simulink model "dc_motor"  (R2025a)
settings: Solver=ode45  StartTime=0.0  StopTime=2  RelTol=1e-3
InitFcn:
  | motor_parameters;
values from neighbouring files (symbols this model uses):
  b = 1e-4    (= 0.0001)    [motor_parameters.m]
  J = 1e-4    (= 0.0001)    [motor_parameters.m]
  Ke = 0.05    [motor_parameters.m]
  Kt = 0.05    [motor_parameters.m]
  L = 0.005    [motor_parameters.m]
  R = 2.0    (= 2)    [motor_parameters.m]
  T_load = 0.01    [motor_parameters.m]
  T_step_time = 0.5    [motor_parameters.m]
  Ts_plant = 0.001    [motor_parameters.m]
  V_step_time = 0.1    [motor_parameters.m]
  V_supply = 6.0    (= 6)    [motor_parameters.m]
undefined symbols (not defined in the file or in its folder): DiscIntNeverNeededParam
settings Model: Creator=quan  LastModifiedBy=quan

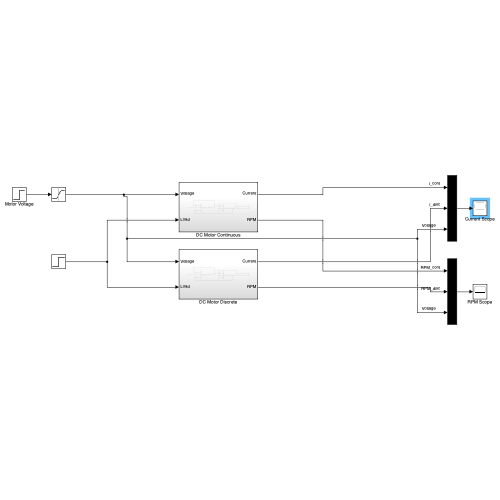
[thumbnail: Simulink's stored preview of the top-level diagram]
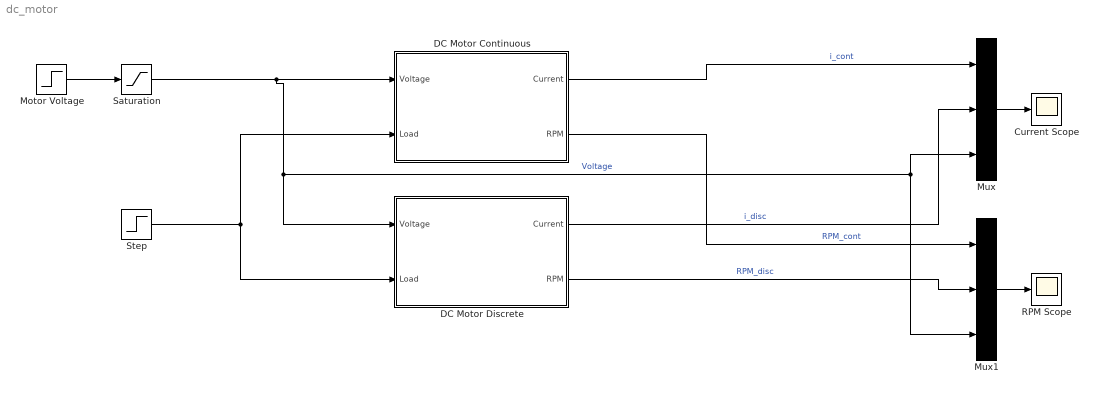
== system dc_motor ==
  Current Scope : Scope
      settings: ActiveDisplayYMinimum=-1.0771917060089902  ActiveDisplayYMaximum=8.4478569944209756
  DC Motor Continuous : Subsystem
  DC Motor Discrete : Subsystem
  Motor Voltage : Step  Time=V_step_time  After=6  SampleTime=0
  Mux : Mux  Inputs=3
  Mux1 : Mux  Inputs=3
  RPM Scope : Scope
      settings: ActiveDisplayYMinimum=701.853464884689  ActiveDisplayYMaximum=780.559508682082
  Saturation : Saturate  UpperLimit=V_supply  LowerLimit=-V_supply
  Step : Step  Time=T_step_time  After=T_load  SampleTime=0
  wires:
  Motor Voltage/1 -> Saturation/1
  Mux/1 -> Current Scope/1
  Saturation/1 -> DC Motor Discrete/1(Voltage), Mux1/3, Mux/3, DC Motor Continuous/1(Voltage)  "Voltage"
  Step/1 -> DC Motor Continuous/2(Load), DC Motor Discrete/2(Load)
  DC Motor Continuous/1(Current) -> Mux/1  "i_cont"
  DC Motor Continuous/2(RPM) -> Mux1/1  "RPM_cont"
  DC Motor Discrete/1(Current) -> Mux/2  "i_disc"
  DC Motor Discrete/2(RPM) -> Mux1/2  "RPM_disc"
  Mux1/1 -> RPM Scope/1

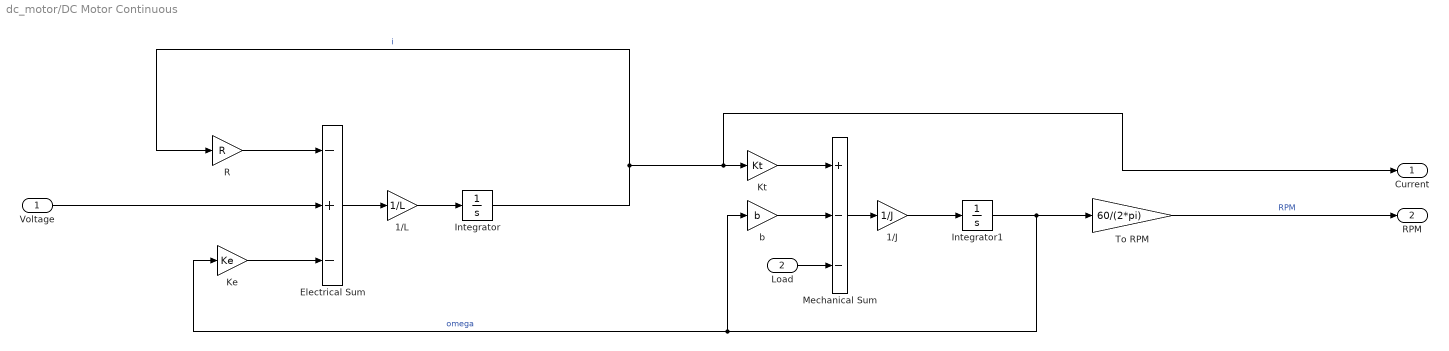
== system dc_motor/DC Motor Continuous ==
  Voltage : Inport
  Load : Inport  Port=2
  1/J : Gain  Gain=1/J
  1/L : Gain  Gain=1/L
  Electrical Sum : Sum  Inputs=-+-
  Integrator : Integrator
  Integrator1 : Integrator
  Ke : Gain  Gain=Ke
  Kt : Gain  Gain=Kt
  Mechanical Sum : Sum  Inputs=+--
  R : Gain  Gain=R
  To RPM : Gain  Gain=60/(2*pi)
  b : Gain  Gain=b
  Current : Outport
  RPM : Outport  Port=2
  wires:
  Ke/1 -> Electrical Sum/3
  b/1 -> Mechanical Sum/2
  Voltage/1 -> Electrical Sum/2
  Integrator1/1 -> Ke/1, b/1, To RPM/1  "omega"
  Mechanical Sum/1 -> 1/J/1
  R/1 -> Electrical Sum/1
  1/L/1 -> Integrator/1
  Electrical Sum/1 -> 1/L/1
  1/J/1 -> Integrator1/1
  Load/1 -> Mechanical Sum/3
  Kt/1 -> Mechanical Sum/1
  To RPM/1 -> RPM/1  "RPM"
  Integrator/1 -> Current/1, Kt/1, R/1  "i"

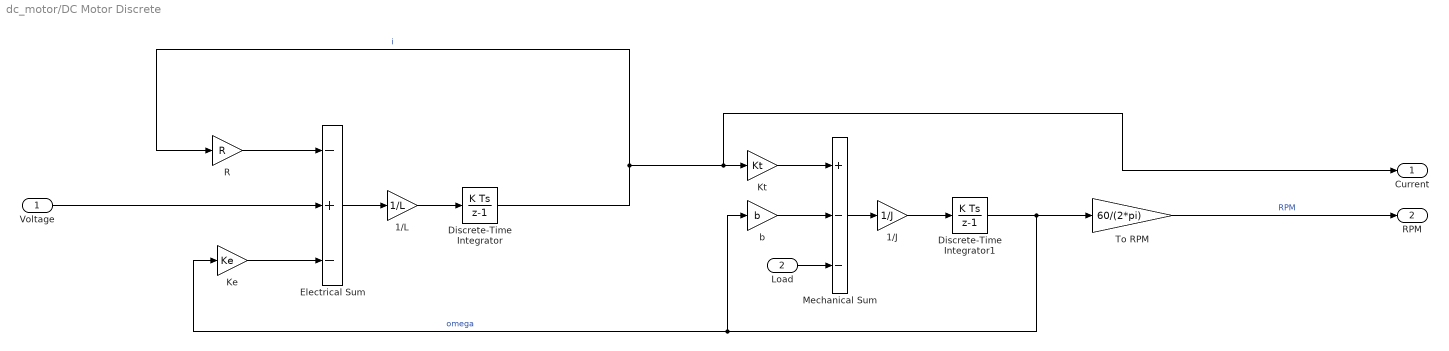
== system dc_motor/DC Motor Discrete ==
  Voltage : Inport
  Load : Inport  Port=2
  1/J : Gain  Gain=1/J
  1/L : Gain  Gain=1/L
  Discrete-Time Integrator : DiscreteIntegrator  SampleTime=Ts_plant  ICPrevOutput=DiscIntNeverNeededParam  ICPrevScaledInput=DiscIntNeverNeededParam
  Discrete-Time Integrator1 : DiscreteIntegrator  SampleTime=Ts_plant  ICPrevOutput=DiscIntNeverNeededParam  ICPrevScaledInput=DiscIntNeverNeededParam
  Electrical Sum : Sum  Inputs=-+-
  Ke : Gain  Gain=Ke
  Kt : Gain  Gain=Kt
  Mechanical Sum : Sum  Inputs=+--
  R : Gain  Gain=R
  To RPM : Gain  Gain=60/(2*pi)
  b : Gain  Gain=b
  Current : Outport
  RPM : Outport  Port=2
  wires:
  Ke/1 -> Electrical Sum/3
  b/1 -> Mechanical Sum/2
  Voltage/1 -> Electrical Sum/2
  Discrete-Time Integrator1/1 -> Ke/1, b/1, To RPM/1  "omega"
  Mechanical Sum/1 -> 1/J/1
  R/1 -> Electrical Sum/1
  1/L/1 -> Discrete-Time Integrator/1
  Electrical Sum/1 -> 1/L/1
  1/J/1 -> Discrete-Time Integrator1/1
  Load/1 -> Mechanical Sum/3
  Kt/1 -> Mechanical Sum/1
  To RPM/1 -> RPM/1  "RPM"
  Discrete-Time Integrator/1 -> Current/1, Kt/1, R/1  "i"
